simulink model "StateEstimator_project"  (R2025b)
settings: Solver=FixedStepAuto  StartTime=0.0  StopTime=2  FixedStep=0.05  RelTol=1e-3
values from neighbouring files (symbols this model uses):
  A_b = [0 1 0 0; num21_a/Z num22_a/(R*Z) 0 num24_a/(R*r*Z) ; 0 0 0 1; num41_a/Z num42_a/(R*Z) 0 num44_a/(R*Z)]    [Project.m]    (also in Project_Jayce.m = double(vpa(A_b,14)); Project_template.m = [])
  B_b = [0; num2_b/den1_b ; 0; num4_b/den1_b]    [Project.m]    (also in Project_Jayce.m = double(vpa(B_b,14)); Project_template.m = [])
  C_b = [1 0 0 0; 0 1 0 0; 0 0 1 0; 0 0 0 1]    [Project.m]    (also in Project_Jayce.m = eye(size(A_b)); Project_template.m = [])
  D_b = [0; 0; 0; 0]    [Project.m]    (also in Project_Jayce.m = [0;0;0;0]; Project_template.m = [])
  L = 0.197    [Project.m]    (also in Project_Jayce.m = place(A_b', C_b', desiredPoles)')
settings Model: Creator=jboar  LastModifiedBy=jboar
settings DataIOCC: SaveFormat=Array  ReturnWorkspaceOutputs=off

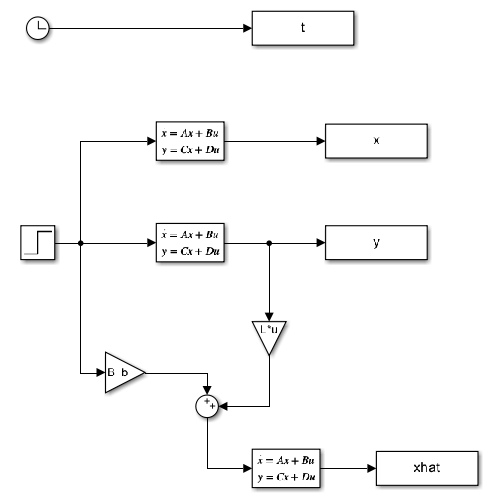
[thumbnail: Simulink's stored preview of the top-level diagram]
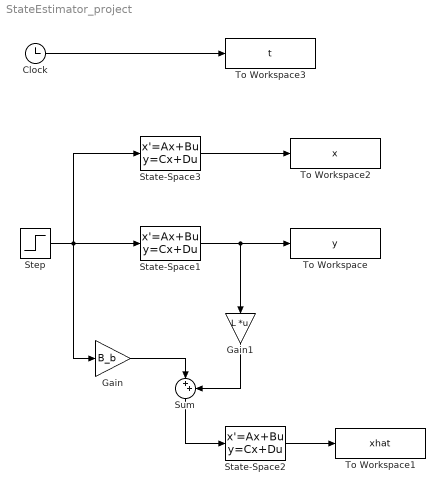
== system StateEstimator_project ==
  Clock : Clock
  Gain : Gain  Gain=B_b
  Gain1 : Gain  Gain=L  Multiplication=Matrix(K*u)
  State-Space1 : StateSpace  A=A_b  B=B_b  C=C_b  D=D_b  InitialCondition=0
  State-Space2 : StateSpace  A=A_b - L*C_b  B=eye(4)  C=eye(4)  D=zeros(4,4)  InitialCondition=0
  State-Space3 : StateSpace  A=A_b  B=B_b  C=eye(size(A_b))  D=zeros(size(C_b, 1),size(B_b,2))  InitialCondition=0
  Step : Step  SampleTime=0
  Sum : Sum  Inputs=|++
  To Workspace : ToWorkspace  VariableName=y  SampleTime=-1
  To Workspace1 : ToWorkspace  VariableName=xhat  SampleTime=-1
  To Workspace2 : ToWorkspace  VariableName=x  SampleTime=-1
  To Workspace3 : ToWorkspace  VariableName=t  SampleTime=-1
  wires:
  Step/1 -> State-Space3/1, Gain/1, State-Space1/1
  State-Space1/1 -> To Workspace/1, Gain1/1
  Gain1/1 -> Sum/2
  Gain/1 -> Sum/1
  Sum/1 -> State-Space2/1
  State-Space2/1 -> To Workspace1/1
  State-Space3/1 -> To Workspace2/1
  Clock/1 -> To Workspace3/1
